simulink model "racketballrev"  (Simulink 7.0)
settings: Solver=FixedStepDiscrete  StartTime=0.0  StopTime=6.0  RelTol=1e-3
undefined symbols (not defined in the file or in its folder): dfilt
libraries: simulink x5, dsparch4 x2, dspwin32 x2
settings Model: Creator=dcs5  LastModifiedBy=dcs5

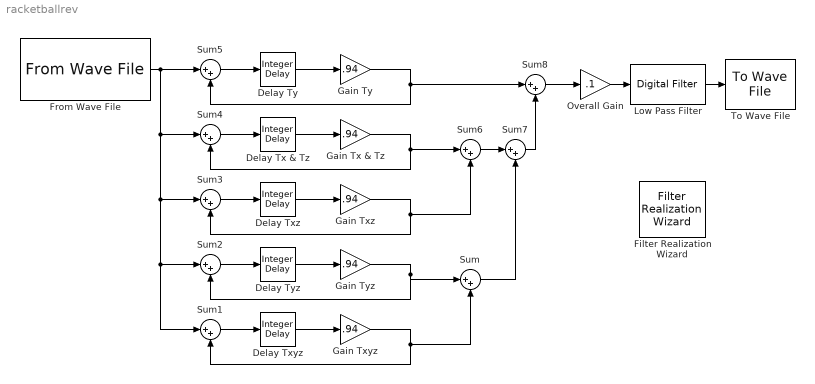
== system racketballrev ==
  Delay Tx & Tz : simulink/Discrete/Integer Delay  vinit=0  samptime=-1  NumDelays=1564
  Delay Txyz : simulink/Discrete/Integer Delay  vinit=0  samptime=-1  NumDelays=3831
  Delay Txz : simulink/Discrete/Integer Delay  vinit=0  samptime=-1  NumDelays=2252
  Delay Ty : simulink/Discrete/Integer Delay  vinit=0  samptime=-1  NumDelays=3128
  Delay Tyz : simulink/Discrete/Integer Delay  vinit=0  samptime=-1  NumDelays=3497
  Filter Realization Wizard : dsparch4/Filter Realization Wizard  SystemSampleTime=-1
  From Wave File : dspwin32/From Wave File  FileName=testing123dry.wav  SamplesPerFrame=1  MinBufSize=1  dType=double  bLoop=off  timesToPlay=1  restartMode=immediately after last sample  firstSampleOutput=off  lastSampleOutput=off
  Gain Tx & Tz : Gain  Gain=.94  ParameterDataType=sfix(16)  ParameterScaling=2^0  OutDataType=sfix(16)  OutScaling=2^0
  Gain Txyz : Gain  Gain=.94  ParameterDataType=sfix(16)  ParameterScaling=2^0  OutDataType=sfix(16)  OutScaling=2^0
  Gain Txz : Gain  Gain=.94  ParameterDataType=sfix(16)  ParameterScaling=2^0  OutDataType=sfix(16)  OutScaling=2^0
  Gain Ty : Gain  Gain=.94  ParameterDataType=sfix(16)  ParameterScaling=2^0  OutDataType=sfix(16)  OutScaling=2^0
  Gain Tyz : Gain  Gain=.94  ParameterDataType=sfix(16)  ParameterScaling=2^0  OutDataType=sfix(16)  OutScaling=2^0
  Low Pass Filter : dsparch4/Digital Filter  Tag=BlockMethodSubSystem  DialogController=dspdialog.DigitalFilter  DialogControllerArgs=DataTag0  TypePopup=IIR (poles & zeros)  IIRFiltStruct=Biquad direct form II (SOS)  AllPoleFiltStruct=Direct form  FIRFiltStruct=Direct form  CoeffSource=Specify via dialog  NumCoeffs=[1 2]  DenCoeffs=[1 0.1]  BiQuadCoeffs=[1 1.48904167641087 1 1 -1.44965219109555 0.534916938247421;1 0.158017147118546 0.999999999999997 1 -1.68378282485485 0.78080102136729]  LatticeCoeffs=[0.2 0.4]  denIgnore=on  FiltPerSampPopup=One filter per frame  IC=0  ICnum=0  ICden=0  roundingMode=Floor  overflowMode=off  ScaleValues=[0.00109865581180459;1;1]  scaleValueFracLength=14  stageInFracLength=15  stageOutFracLength=15  FilterSource=Specify via dialog  dfiltObjectName=dfilt.dffir([1 2 1])
  Overall Gain : Gain  Gain=.1  ParameterDataType=sfix(16)  ParameterScaling=2^0  OutDataType=sfix(16)  OutScaling=2^0
  Sum{,1..8} (9 alike) : Sum  Inputs=|++  OutDataType=sfix(16)  OutScaling=2^0
  To Wave File : dspwin32/To Wave File  filename=audio  sampleWidth=16  MinNumSamples=256
  wires:
  Delay Txyz/1 -> Gain Txyz/1
  Gain Txyz/1 -> Sum1/2, Sum/2
  Sum1/1 -> Delay Txyz/1
  Delay Tyz/1 -> Gain Tyz/1
  Gain Tyz/1 -> Sum2/2, Sum/1
  Sum2/1 -> Delay Tyz/1
  Delay Txz/1 -> Gain Txz/1
  Gain Txz/1 -> Sum3/2, Sum6/2
  Sum3/1 -> Delay Txz/1
  Delay Tx & Tz/1 -> Gain Tx & Tz/1
  Gain Tx & Tz/1 -> Sum4/2, Sum6/1
  Sum4/1 -> Delay Tx & Tz/1
  Delay Ty/1 -> Gain Ty/1
  Gain Ty/1 -> Sum5/2, Sum8/1
  Sum5/1 -> Delay Ty/1
  Sum6/1 -> Sum7/1
  Sum/1 -> Sum7/2
  Sum7/1 -> Sum8/2
  From Wave File/1 -> Sum5/1, Sum4/1, Sum3/1, Sum2/1, Sum1/1
  Sum8/1 -> Overall Gain/1
  Overall Gain/1 -> Low Pass Filter/1
  Low Pass Filter/1 -> To Wave File/1
